simulink model "import_kernel"  (R2020a)
settings: Solver=VariableStepAuto  StartTime=0.0  StopTime=32*128 - 1  RelTol=1e-3
InitFcn:
  | xmcCheckSlxPath(bdroot);
  | input = readcomplexdata('input.txt');
  | assignin('base', 'input', input);
libraries: dspsrcs4 x1
settings Model: Creator=jou  LastModifiedBy=viswanad
settings DataIOCC: ReturnWorkspaceOutputs=off
settings DebuggingCC: PregeneratedLibrarySubsystemCodeDiagnostic=none  ArithmeticOperatorsInVariantConditions=warning
settings SFSimCC: SimUseLocalCustomCode=off  CustomCodeUndefinedFunction=UseInterfaceOnly
settings RTWCC: RTWUseLocalCustomCode=off

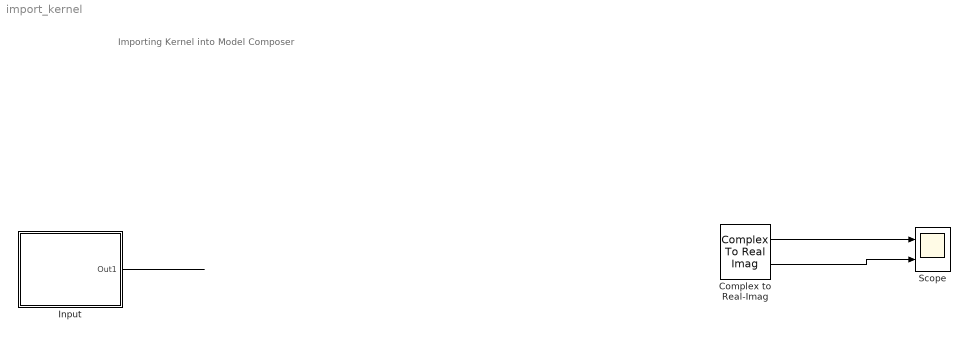
== system import_kernel ==
  note: Importing Kernel into Model Composer
  Complex to Real-Imag : ComplexToRealImag
  Input : Subsystem
  Scope : Scope  NumInputPorts=2
  wires:
  Complex to Real-Imag/1 -> Scope/1
  Complex to Real-Imag/2 -> Scope/2
  Input/1(Out1) -> ?
  ? -> Complex to Real-Imag/1

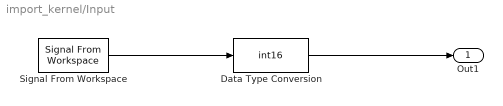
== system import_kernel/Input ==
  Data Type Conversion : DataTypeConversion  OutDataTypeStr=int16
  Signal From Workspace : dspsrcs4/Signal From Workspace  X=input  Ts=1  nsamps=128  OutputAfterFinalValue=Setting to zero  ignoreOrWarnInputAndFrameLengths=off  OutputFrames=off
  Out1 : Outport  VectorParamsAs1DForOutWhenUnconnected=off
  wires:
  Signal From Workspace/1 -> Data Type Conversion/1
  Data Type Conversion/1 -> Out1/1
